simulink library "NewtonEuler_Lib"  (R2024b)
settings: Solver=VariableStepAuto  StartTime=0.0  StopTime=10.0  RelTol=1e-3
settings Model: Creator=pepev  LastModifiedBy=pepev

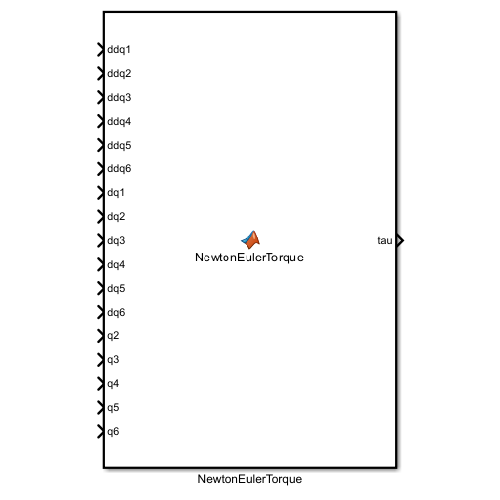
[thumbnail: Simulink's stored preview of the top-level diagram]
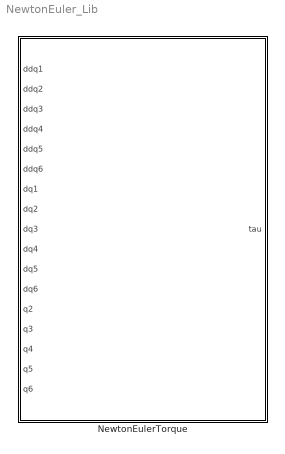
== system NewtonEuler_Lib ==
  NewtonEulerTorque : MATLAB Function  TreatAsAtomicUnit=on

== matlab function NewtonEuler_Lib/NewtonEulerTorque ==
  data: ddq1 input; tau output; ddq2 input; ddq3 input; ddq4 input; ddq5 input; ddq6 input; dq1 input; dq2 input; dq3 input; dq4 input; dq5 input; dq6 input; q2 input; q3 input; q4 input; q5 input; q6 input
function tau = NewtonEulerTorque(ddq1,ddq2,ddq3,ddq4,ddq5,ddq6,dq1,dq2,dq3,dq4,dq5,dq6,q2,q3,q4,q5,q6)
%#codegen

%    This function was generated by the Symbolic Math Toolbox version 24.2.
%    17-Jun-2025 17:09:40

% ddq1 = complex(ddq1);  % if required to enforce complex operations
% ddq2 = complex(ddq2);  % if required to enforce complex operations
% ddq3 = complex(ddq3);  % if required to enforce complex operations
% ddq4 = complex(ddq4);  % if required to enforce complex operations
% ddq5 = complex(ddq5);  % if required to enforce complex operations
% ddq6 = complex(ddq6);  % if required to enforce complex operations
% dq1 = complex(dq1);  % if required to enforce complex operations
% dq2 = complex(dq2);  % if required to enforce complex operations
% dq3 = complex(dq3);  % if required to enforce complex operations
% dq4 = complex(dq4);  % if required to enforce complex operations
% dq5 = complex(dq5);  % if required to enforce complex operations
% dq6 = complex(dq6);  % if required to enforce complex operations
% q2 = complex(q2);  % if required to enforce complex operations
% q3 = complex(q3);  % if required to enforce complex operations
% q4 = complex(q4);  % if required to enforce complex operations
% q5 = complex(q5);  % if required to enforce complex operations
% q6 = complex(q6);  % if required to enforce complex operations
t2 = cos(q2);
t3 = cos(q3);
t4 = cos(q4);
t5 = cos(q5);
t6 = cos(q6);
t7 = sin(q2);
t8 = sin(q3);
t9 = sin(q4);
t10 = sin(q5);
t11 = sin(q6);
t12 = dq2.*dq3;
t20 = -ddq3;
t21 = -ddq5;
t23 = sqrt(2.0);
t34 = ddq4./2.0e+2;
t35 = dq4./2.0e+2;
t44 = ddq3.*4.375e-3;
t45 = dq3.*4.375e-3;
t78 = ddq5.*6.3175e-2;
t79 = dq5.*6.3175e-2;
t13 = t4.^2;
t14 = t9.^2;
t15 = ddq1.*t2;
t16 = dq2.*t3;
t17 = ddq1.*t7;
t18 = dq1.*t7;
t19 = dq2.*t8;
t24 = dq1.*dq2.*t2;
t25 = dq1.*dq3.*t2;
t26 = dq1.*t2.*t3;
t27 = dq1.*t2.*t8;
t32 = t23+2.0;
t43 = -t23;
t66 = t7.*(9.81e+2./1.0e+2);
t81 = t2.*t3.*(9.81e+2./1.0e+2);
t82 = t2.*t3.*2.943e+1;
t83 = t2.*t8.*(9.81e+2./1.0e+2);
t94 = t2.*t3.*4.4145;
t22 = dq2.*t18;
t28 = -t15;
t29 = -t17;
t30 = -t18;
t31 = -t19;
t33 = ddq2+t25;
t36 = -t24;
t38 = -t26;
t39 = t15.*(3.0./1.0e+1);
t40 = t16.*(3.0./1.0e+1);
t41 = t17.*(3.0./1.0e+1);
t42 = t19.*(3.0./1.0e+1);
t47 = t13./1.0e+1;
t49 = t15.*(9.0./1.0e+1);
t50 = t14./1.0e+1;
t51 = t19./2.0e+2;
t52 = t24.*(3.0./1.0e+1);
t55 = t43+2.0;
t57 = t26.*(3.0./1.0e+1);
t58 = t27.*(3.0./1.0e+1);
t60 = t15.*(2.7e+1./2.0e+2);
t62 = t18.*4.375e-3;
t65 = sqrt(t32);
t68 = t26./2.0e+2;
t69 = t16+t27;
t75 = -t66;
t76 = t16.*2.84375e-2;
t77 = t19.*2.84375e-2;
t87 = t26.*2.84375e-2;
t88 = t27.*2.84375e-2;
t92 = t17+t20+t24;
t37 = dq3+t30;
t46 = t22.*(3.0./1.0e+1);
t53 = t8.*t33;
t54 = t22.*(9.0./1.0e+1);
t61 = -t51;
t63 = t3.*t33;
t64 = t22.*(2.7e+1./2.0e+2);
t67 = -t57;
t72 = -t62;
t84 = dq4.*t69;
t85 = t19+t38;
t89 = sqrt(t55);
t90 = t4.*t69;
t91 = t9.*t69;
t93 = dq4+t26+t31;
t95 = t12+t22+t28;
t96 = -t87;
t109 = t40+t58;
t110 = t47+t50;
t130 = t76+t88;
t56 = dq4.*t37;
t71 = t4.*t37;
t73 = t9.*t37;
t74 = -t53;
t80 = -t63;
t97 = t93.^2;
t98 = dq5.*t93;
t101 = t5.*t93;
t102 = t10.*t93;
t104 = t53.*3.34375e-2;
t105 = t3.*t95;
t106 = t8.*t95;
t107 = t63.*2.84375e-2;
t111 = t90./2.0e+2;
t112 = t91./2.0e+2;
t118 = t42+t67;
t119 = t45+t72;
t122 = t90.*6.3175e-2;
t131 = t37.*t109;
t132 = t77+t96;
t134 = ddq3+t29+t36+t84;
t137 = t35+t61+t68;
t145 = t69.*t109;
t165 = t92.*t110;
t172 = t37.*t130;
t187 = t85.*t130;
t86 = -t73;
t99 = t71./2.0e+2;
t100 = t73./2.0e+2;
t108 = -t104;
t113 = t101./2.0;
t114 = t101./4.0;
t115 = t102./2.0;
t116 = t102./4.0;
t117 = -t105;
t120 = t73.*6.3175e-2;
t123 = t101.*1.35e-3;
t124 = t105.*3.34375e-2;
t125 = t106.*2.84375e-2;
t126 = t71+t91;
t127 = t102.*6.3175e-2;
t138 = t37.*t118;
t139 = t53+t105;
t142 = (t73-t90).^2;
t143 = -t131;
t146 = t4.*t134;
t148 = t9.*t134;
t151 = t69.*t119;
t162 = t85.*t118;
t163 = t85.*t119;
t170 = t165.*6.0;
t171 = t97.*t110;
t179 = t37.*t132;
t185 = t69.*t132;
t189 = t56+t80+t106;
t234 = t137.*(t73-t90);
t103 = -t100;
t121 = -t120;
t128 = -t124;
t133 = dq5.*t126;
t135 = t86+t90;
t140 = t5.*t126;
t141 = t10.*t126;
t144 = t138.*3.0;
t156 = -t146;
t158 = -t148;
t161 = t138.*(9.0./2.0e+1);
t164 = -t151;
t166 = t146./2.0;
t167 = t146.*(3.0./2.0);
t168 = t148./2.0;
t169 = t148.*(3.0./2.0);
t174 = t99+t112;
t177 = t146./2.0e+2;
t178 = t171.*3.0;
t188 = t148.*6.8175e-2;
t191 = t4.*t189;
t192 = t9.*t189;
t205 = t110.*t139;
t207 = t110.*t142;
t228 = t126.*t137;
t235 = t93.*t110.*t126;
t236 = t41+t52+t83+t143;
t273 = t75+t145+t162;
t136 = dq5+t135;
t149 = -t140;
t152 = t140./2.0;
t153 = t140./4.0;
t154 = t141./2.0;
t155 = t141./4.0;
t180 = t103+t111;
t181 = -t177;
t182 = t141.*1.35e-3;
t184 = t140.*6.3175e-2;
t193 = -t191;
t195 = t191./2.0;
t196 = t191.*(3.0./2.0);
t197 = t192./2.0;
t198 = t192.*(3.0./2.0);
t199 = t101+t141;
t203 = t192./2.0e+2;
t208 = t205.*3.0;
t210 = t207.*3.0;
t214 = t93.*t174;
t220 = t191.*6.8175e-2;
t223 = t205.*(9.0./2.0e+1);
t233 = t79+t121+t122;
t237 = t235.*3.0;
t240 = ddq4+t74+t117+t133;
t243 = t4.*t236;
t244 = t9.*t236;
t246 = t235.*(9.0./2.0e+1);
t259 = t174.*(t73-t90);
t275 = t21+t148+t191;
t276 = t4.*t273;
t277 = t9.*t273;
t293 = t98+t156+t192;
t340 = -t5.*(t39-t46-t81-t138+t205+t235);
t342 = t5.*(t39-t46-t81-t138+t205+t235).*-3.0;
t345 = t10.*(t39-t46-t81-t138+t205+t235);
t147 = dq6.*t136;
t150 = t6.*t136;
t159 = -t152;
t160 = -t153;
t186 = -t184;
t194 = (t11.*t65.*t136)./2.0;
t200 = -t197;
t201 = -t198;
t202 = dq6+t199;
t204 = t102+t149;
t206 = (t11.*t89.*t136)./2.0;
t216 = t93.*t180;
t217 = t113+t154;
t218 = t114+t155;
t219 = t11.*t89.*t136.*(2.3e+1./8.0e+2);
t227 = t11.*t89.*t136.*5.625e-5;
t242 = t123+t182;
t245 = t126.*t180;
t247 = t243.*6.0;
t248 = t244.*3.0;
t250 = t5.*t240;
t251 = t10.*t240;
t274 = t11.*t65.*t136.*5.791666666666666e-4;
t278 = t276.*3.0;
t279 = t277.*6.0;
t295 = t5.*t293;
t296 = t10.*t293;
t299 = (t89.*t275)./2.0e+1;
t308 = t89.*t275.*2.875e-3;
t322 = t199.*t233;
t346 = t345.*3.0;
t368 = t171+t207+t244+t276;
t157 = -t147;
t183 = t150.*(2.3e+1./4.0e+2);
t209 = -t206;
t211 = dq6.*t204;
t215 = t11.*t204;
t221 = t115+t159;
t222 = t116+t160;
t224 = -t219;
t229 = -t227;
t241 = (t65.*t202)./2.0;
t255 = (t89.*t202)./2.0;
t256 = (t6.*t65.*t204)./2.0;
t257 = t65.*t202.*(2.3e+1./8.0e+2);
t261 = t150.*1.158333333333333e-3;
t262 = t127+t186;
t263 = t250.*(3.0./4.0);
t264 = t251.*(3.0./4.0);
t265 = (t6.*t89.*t204)./2.0;
t266 = t65.*t202.*5.625e-5;
t267 = t6.*t89.*t204.*(2.3e+1./8.0e+2);
t268 = t250.*1.35e-3;
t270 = t6.*t89.*t204.*5.625e-5;
t272 = t251.*6.3175e-2;
t280 = t136.*t217;
t283 = t136.*t218.*3.0;
t292 = t136.*t242;
t300 = -t296;
t301 = t89.*t202.*5.791666666666666e-4;
t302 = t6.*t65.*t204.*5.791666666666666e-4;
t303 = t295.*(3.0./4.0);
t304 = t296.*(3.0./4.0);
t306 = t199.*t217;
t310 = t199.*t218.*3.0;
t316 = t296.*1.35e-3;
t321 = t295.*6.3175e-2;
t323 = t204.*t233;
t325 = t204.*t242;
t335 = t251+t295;
t369 = t5.*t368;
t370 = t10.*t368;
t232 = t215.*(2.3e+1./4.0e+2);
t258 = -t256;
t281 = t136.*t221;
t282 = t280.*3.0;
t284 = t150+t215;
t286 = -t283;
t287 = t136.*t222.*3.0;
t291 = t215.*1.158333333333333e-3;
t294 = -t292;
t298 = t136.*t262;
t305 = -t302;
t307 = -t304;
t309 = t306.*3.0;
t313 = t204.*t221;
t315 = t204.*t222.*3.0;
t319 = -t316;
t324 = -t323;
t326 = t199.*t262;
t328 = ddq5+t158+t193+t211;
t337 = ddq6+t250+t300;
t344 = (t65.*t335)./2.0e+1;
t349 = t65.*(t250+t300).*(-1.0./2.0e+1);
t351 = (t89.*t335)./2.0e+1;
t353 = t209+t241+t265;
t354 = t65.*(t250+t300).*(-2.875e-3);
t355 = t89.*t335.*2.875e-3;
t358 = t224+t257+t267;
t359 = t157+t335;
t362 = t229+t266+t270;
t371 = t369.*3.0;
t372 = t370.*3.0;
t405 = t166+t200+t280+t340+t370;
t285 = t281.*3.0;
t288 = -t281;
t290 = t284.^2;
t297 = t183+t232;
t314 = t313.*3.0;
t327 = -t326;
t329 = t6.*t328.*(2.3e+1./4.0e+2);
t330 = t11.*t89.*t328.*(2.3e+1./8.0e+2);
t332 = t261+t291;
t333 = t11.*t89.*t328.*1.709375e-3;
t339 = t6.*t328.*4.464583333333333e-3;
t347 = -t344;
t348 = t194+t255+t258;
t350 = t11.*t65.*t328.*5.791666666666666e-4;
t356 = t65.*t337.*(2.3e+1./8.0e+2);
t357 = t65.*t337.*1.709375e-3;
t363 = (t89.*t353)./2.0e+1;
t364 = t11.*t359.*(2.3e+1./4.0e+2);
t365 = t89.*t337.*5.791666666666666e-4;
t366 = t6.*t89.*t359.*(2.3e+1./8.0e+2);
t367 = t6.*t89.*t359.*1.709375e-3;
t373 = t11.*t359.*4.464583333333333e-3;
t374 = t6.*t65.*t359.*5.791666666666666e-4;
t377 = t274+t301+t305;
t378 = (t65.*t284.*t353)./2.0e+1;
t381 = t284.*t362;
t382 = t65.*t284.*t353.*2.875e-3;
t391 = t353.*t358;
t399 = -t6.*(t165+t243-t277-t306-t313+t110.*t126.*(t73-t90));
t400 = t6.*(t165+t243-t277-t306-t313+t110.*t126.*(t73-t90)).*(-2.3e+1./4.0e+2);
t402 = (t11.*t65.*(t165+t243-t277-t306-t313+t110.*t126.*(t73-t90)))./2.0;
t403 = t11.*t89.*(t165+t243-t277-t306-t313+t110.*t126.*(t73-t90)).*(-1.0./2.0);
t404 = t11.*t89.*(t165+t243-t277-t306-t313+t110.*t126.*(t73-t90)).*(-2.3e+1./8.0e+2);
t414 = (t65.*t405)./2.0;
t415 = (t89.*t405)./2.0;
t416 = t65.*t405.*(2.3e+1./8.0e+2);
t289 = -t285;
t312 = (t65.*t290)./2.0e+1;
t318 = t65.*t290.*2.875e-3;
t320 = (t89.*t290)./2.0e+1;
t331 = -t330;
t334 = -t333;
t352 = t284.*t297;
t360 = (t65.*t348)./2.0e+1;
t375 = -t374;
t376 = t297.*t348;
t379 = (t89.*t284.*t348)./2.0e+1;
t383 = t89.*t284.*t348.*2.875e-3;
t384 = t332.*t348;
t385 = t332.*t353;
t387 = t284.*t377;
t389 = t348.*t358;
t393 = t348.*t362;
t397 = t353.*t377;
t407 = t168+t195+t288+t345+t369;
t380 = t376.*(2.3e+1./4.0e+2);
t386 = -t385;
t388 = -t387;
t390 = -t389;
t392 = t389.*(2.3e+1./4.0e+2);
t395 = -t393;
t408 = t348.*(t360-t363);
t409 = -t353.*(t360-t363);
t410 = t11.*t407;
t417 = (t6.*t65.*t407)./2.0;
t418 = (t6.*t89.*t407)./2.0;
t420 = t6.*t89.*t407.*(2.3e+1./8.0e+2);
t394 = -t392;
t412 = t408.*(2.3e+1./4.0e+2);
t413 = t410.*(2.3e+1./4.0e+2);
t419 = -t418;
t421 = -t420;
t422 = t350+t365+t375+t381+t386;
t427 = t299+t331+t349+t356+t366+t376+t378+t379+t399+t410;
t432 = t320+t347+t352+t391+t402+t409+t415+t417;
t423 = (t11.*t65.*t422)./2.0;
t424 = (t6.*t65.*t422)./2.0;
t425 = (t89.*t422)./2.0;
t428 = t6.*t427;
t429 = t11.*t427;
t433 = (t6.*t65.*t432)./2.0;
t434 = (t11.*t65.*t432)./2.0;
t435 = (t6.*t65.*t432)./8.0;
t437 = (t89.*t432)./2.0;
t439 = (t89.*t432)./8.0;
t441 = t312+t329+t351+t364+t390+t403+t408+t414+t419;
t449 = t308+t334+t354+t357+t367+t380+t382+t383+t384+t388+t400+t413;
t454 = t318+t339+t355+t373+t394+t395+t397+t404+t412+t416+t421;
t426 = -t424;
t430 = t429./4.0;
t438 = -t435;
t440 = -t439;
t442 = (t65.*t441)./2.0;
t443 = (t65.*t441)./8.0;
t445 = (t6.*t89.*t441)./2.0;
t446 = (t11.*t89.*t441)./2.0;
t448 = (t6.*t89.*t441)./8.0;
t450 = (t65.*t449)./2.0;
t451 = (t6.*t89.*t449)./2.0;
t452 = (t11.*t89.*t449)./2.0;
t455 = t6.*t454;
t456 = t11.*t454;
t431 = -t430;
t444 = -t443;
t447 = -t445;
t453 = -t452;
t457 = t167+t201+t264+t282+t286+t303+t342+t372+t437+t442;
t462 = t4.*(t170+t247-t279-t309+t310-t314+t315-t428+t434-t446+t110.*t126.*(t73-t90).*6.0).*(-3.0./2.0e+1);
t463 = -t110.*(t170+t247-t279-t309+t310-t314+t315-t428+t434-t446+t110.*t126.*(t73-t90).*6.0);
t458 = t5.*t457;
t459 = t10.*t457;
t464 = t169+t196+t263+t287+t289+t307+t346+t371+t429+t433+t447;
t470 = t268+t298+t319+t324+t425+t431+t438+t448+t450;
t474 = t272+t294+t321+t322+t426+t440+t444+t451+t456;
t460 = t458.*(3.0./2.0e+1);
t465 = t5.*t464;
t466 = t10.*t464;
t471 = t5.*t470;
t472 = t10.*t470;
t475 = t5.*t474;
t476 = t10.*t474;
t468 = t466.*(3.0./2.0e+1);
t473 = -t472;
t479 = t178+t210+t248+t278+t459+t465;
t484 = -t9.*(-t78+t188-t214+t220+t228-t325+t326-t423+t452-t455+t110.*(t49-t54-t82-t144+t208+t237-t458+t466));
t480 = t9.*t479.*(3.0./2.0e+1);
t485 = t181+t203+t216+t234+t473+t475;
t481 = -t480;
t486 = t4.*t485;
t487 = t9.*t485;
t489 = t34+t108+t128+t164+t172+t245+t259+t462+t463+t471+t476+t481;
mt1 = [ddq1.*(2.7e+1./5.0e+2)+t2.*(t15.*(2.0./1.25e+2)-t22.*(2.0./1.25e+2)-t8.*(t60-t64-t94-t107+t125-t161+t163-t179+t223+t246-t460+t468+t487+t4.*(-t78+t188-t214+t220+t228-t325+t326-t423+t452-t455+t110.*(t49-t54-t82-t144+t208+t237-t458+t466)))+t3.*t489)+t7.*(t17.*2.0375e-2+t24.*2.0375e-2-t44+t185-t187+t484+t486)];
mt2 = [ddq2.*(2.0./1.25e+2)-t3.*(t60-t64-t94-t107+t125-t161+t163-t179+t223+t246-t460+t468+t487+t4.*(-t78+t188-t214+t220+t228-t325+t326-t423+t452-t455+t110.*(t49-t54-t82-t144+t208+t237-t458+t466)))-t8.*t489;t17.*(-4.375e-3)-t24.*4.375e-3+t44-t185+t187-t486+t9.*(-t78+t188-t214+t220+t228-t325+t326-t423+t452-t455+t110.*(t49-t54-t82-t144+t208+t237-t458+t466))];
mt3 = [t34-t53./2.0e+2-t105./2.0e+2+t245+t259+t463+t471+t476;t78-t148.*6.3175e-2-t191.*6.3175e-2+t325+t327+t423+t453+t455;t425+t450];
tau = [mt1;mt2;mt3];
end
